simulink model "TDMA1"  (Simulink 7.6)
settings: Solver=ode45  StartTime=0.0  StopTime=5.0  RelTol=1e-3
settings Model: Creator=matlab  LastModifiedBy=matlab

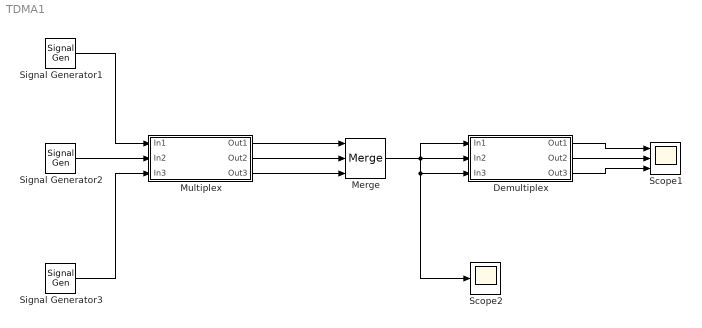
== system TDMA1 ==
  Demultiplex : Subsystem
  Merge : Merge  Inputs=3
  Multiplex : Subsystem
  Scope1 : Scope  NumInputPorts=3
      settings: YMin=-5~-5~-5  YMax=5~5~5
  Scope2 : Scope
  Signal Generator1 : SignalGenerator  Frequency=4
  Signal Generator2 : SignalGenerator  WaveForm=square  Frequency=0.5
  Signal Generator3 : SignalGenerator  WaveForm=sawtooth
  wires:
  Multiplex/1(Out1) -> Merge/1
  Multiplex/2(Out2) -> Merge/2
  Multiplex/3(Out3) -> Merge/3
  Signal Generator1/1 -> Multiplex/1(In1)
  Signal Generator2/1 -> Multiplex/2(In2)
  Signal Generator3/1 -> Multiplex/3(In3)
  Merge/1 -> Scope2/1, Demultiplex/3(In3), Demultiplex/1(In1), Demultiplex/2(In2)
  Demultiplex/1(Out1) -> Scope1/1
  Demultiplex/2(Out2) -> Scope1/2
  Demultiplex/3(Out3) -> Scope1/3

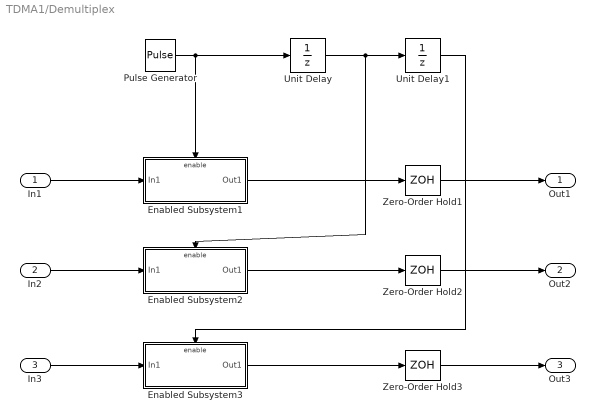
== system TDMA1/Demultiplex ==
  In1 : Inport
  In2 : Inport  Port=2
  In3 : Inport  Port=3
  Enabled Subsystem1 : Subsystem  TreatAsAtomicUnit=on
  Enabled Subsystem2 : Subsystem  TreatAsAtomicUnit=on
  Enabled Subsystem3 : Subsystem  TreatAsAtomicUnit=on
  Pulse Generator : DiscretePulseGenerator  PulseType=Time based  Period=0.003  PulseWidth=100/3
  Unit Delay : UnitDelay  SampleTime=-1
  Unit Delay1 : UnitDelay  SampleTime=-1
  Zero-Order Hold1 : ZeroOrderHold  SampleTime=0.001
  Zero-Order Hold2 : ZeroOrderHold  SampleTime=0.001
  Zero-Order Hold3 : ZeroOrderHold  SampleTime=0.001
  Out1 : Outport
  Out2 : Outport  Port=2
  Out3 : Outport  Port=3
  wires:
  Pulse Generator/1 -> Unit Delay/1, Enabled Subsystem1/Enable
  Unit Delay/1 -> Unit Delay1/1, Enabled Subsystem2/Enable
  Unit Delay1/1 -> Enabled Subsystem3/Enable
  Enabled Subsystem1/1(Out1) -> Zero-Order Hold1/1
  Enabled Subsystem2/1(Out1) -> Zero-Order Hold2/1
  Enabled Subsystem3/1(Out1) -> Zero-Order Hold3/1
  Zero-Order Hold1/1 -> Out1/1
  Zero-Order Hold2/1 -> Out2/1
  Zero-Order Hold3/1 -> Out3/1
  In1/1 -> Enabled Subsystem1/1(In1)
  In2/1 -> Enabled Subsystem2/1(In1)
  In3/1 -> Enabled Subsystem3/1(In1)

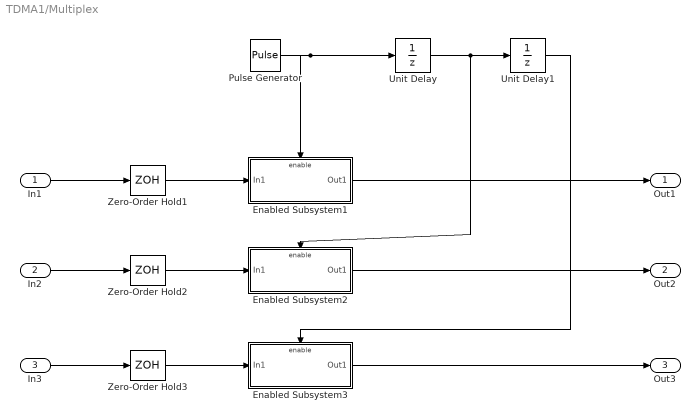
== system TDMA1/Multiplex ==
  In1 : Inport
  In2 : Inport  Port=2
  In3 : Inport  Port=3
  Enabled Subsystem1 : Subsystem  TreatAsAtomicUnit=on
  Enabled Subsystem2 : Subsystem  TreatAsAtomicUnit=on
  Enabled Subsystem3 : Subsystem  TreatAsAtomicUnit=on
  Pulse Generator : DiscretePulseGenerator  PulseType=Time based  Period=0.003  PulseWidth=100/3
  Unit Delay : UnitDelay  SampleTime=-1
  Unit Delay1 : UnitDelay  SampleTime=-1
  Zero-Order Hold1 : ZeroOrderHold  SampleTime=0.001
  Zero-Order Hold2 : ZeroOrderHold  SampleTime=0.001
  Zero-Order Hold3 : ZeroOrderHold  SampleTime=0.001
  Out1 : Outport
  Out2 : Outport  Port=2
  Out3 : Outport  Port=3
  wires:
  Pulse Generator/1 -> Unit Delay/1, Enabled Subsystem1/Enable
  Unit Delay/1 -> Unit Delay1/1, Enabled Subsystem2/Enable
  Unit Delay1/1 -> Enabled Subsystem3/Enable
  Enabled Subsystem1/1(Out1) -> Out1/1
  Enabled Subsystem2/1(Out1) -> Out2/1
  Enabled Subsystem3/1(Out1) -> Out3/1
  Zero-Order Hold3/1 -> Enabled Subsystem3/1(In1)
  In3/1 -> Zero-Order Hold3/1
  Zero-Order Hold2/1 -> Enabled Subsystem2/1(In1)
  In2/1 -> Zero-Order Hold2/1
  Zero-Order Hold1/1 -> Enabled Subsystem1/1(In1)
  In1/1 -> Zero-Order Hold1/1

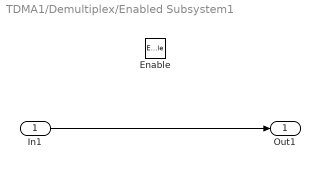
== system TDMA1/Demultiplex/Enabled Subsystem1 ==
  In1 : Inport
  Enable : EnablePort
  Out1 : Outport
  wires:
  In1/1 -> Out1/1

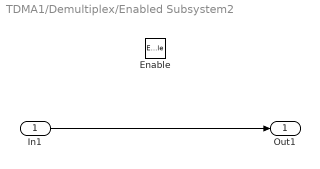
== system TDMA1/Demultiplex/Enabled Subsystem2 ==
  In1 : Inport
  Enable : EnablePort
  Out1 : Outport
  wires:
  In1/1 -> Out1/1

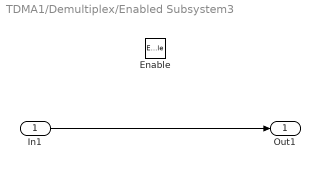
== system TDMA1/Demultiplex/Enabled Subsystem3 ==
  In1 : Inport
  Enable : EnablePort
  Out1 : Outport
  wires:
  In1/1 -> Out1/1

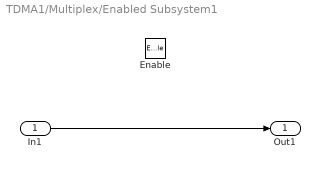
== system TDMA1/Multiplex/Enabled Subsystem1 ==
  In1 : Inport
  Enable : EnablePort
  Out1 : Outport
  wires:
  In1/1 -> Out1/1

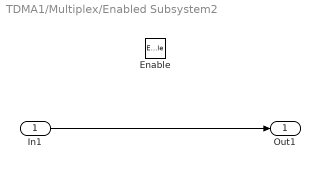
== system TDMA1/Multiplex/Enabled Subsystem2 ==
  In1 : Inport
  Enable : EnablePort
  Out1 : Outport
  wires:
  In1/1 -> Out1/1

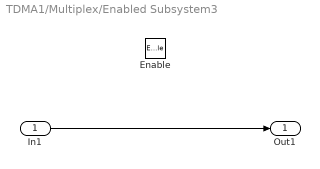
== system TDMA1/Multiplex/Enabled Subsystem3 ==
  In1 : Inport
  Enable : EnablePort
  Out1 : Outport
  wires:
  In1/1 -> Out1/1
